simulink model "Subsystem"  (R2020b)
settings: Solver=VariableStepAuto  StartTime=0.0  StopTime=0.2  RelTol=1e-3
InitFcn:
  | J=3.2284e-6;
  | b=3.5077e-6;
  | Ke= 0.0274;
  | Kt=   0.0274;
  | R=4;
  | L=2.75e-6;
values from neighbouring files (symbols this model uses):
  Kd = 0.058185    [MBD2_problem4_data.sldd]
  Ki = 750.0    [MBD2_problem4_data.sldd]
  Kp = 40.4299    [MBD2_problem4_data.sldd]
settings Model: Creator=Lenovo  LastModifiedBy=Lenovo
settings DataIOCC: SaveOutput=off  SaveTime=off

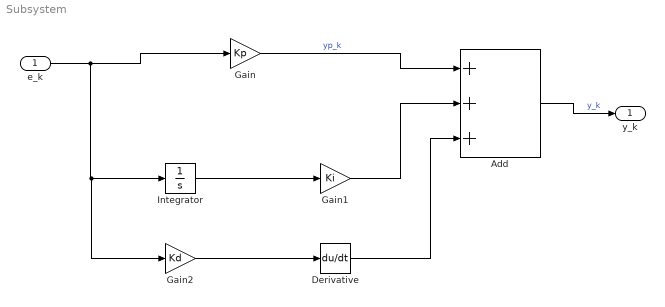
== system Subsystem ==
  e_k : Inport  OutDataTypeStr=double  PortDimensions=1  SampleTime=0
  Add : Sum  Inputs=+++
  Derivative : Derivative
  Gain : Gain  Gain=Kp
  Gain1 : Gain  Gain=Ki
  Gain2 : Gain  Gain=Kd
  Integrator : Integrator
  y_k : Outport  OutDataTypeStr=double  PortDimensions=1  SampleTime=0
  wires:
  Gain2/1 -> Derivative/1
  Derivative/1 -> Add/3
  Add/1 -> y_k/1  "y_k"
  e_k/1 -> Gain/1, Gain2/1, Integrator/1
  Gain1/1 -> Add/2
  Gain/1 -> Add/1  "yp_k"
  Integrator/1 -> Gain1/1
